simulink model "rx"  (R2019a)
settings: Solver=VariableStepAuto  StartTime=0.0  StopTime=10.0  RelTol=1e-3
undefined symbols (not defined in the file): fdesignblkfcn, gcbh
libraries: audiosources x1
settings Model: Creator=vicda  LastModifiedBy=vicda

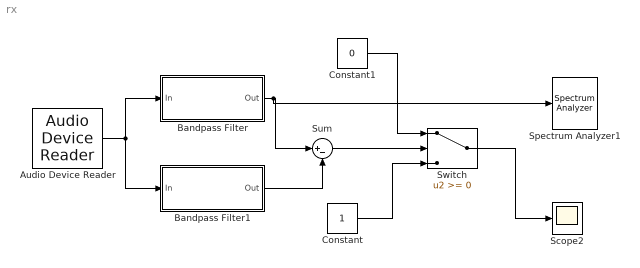
== system rx ==
  Audio Device Reader : audiosources/Audio Device Reader  Driver=DirectSound  Device=Default  SampleRate=44100  NumChannels=1  SamplesPerFrame=512  BitDepth=16-bit integer  NumBuffers=10  DefaultInputChannelMapping=on  InputChannelMapping=1:2  OutputNumOverrunSamples=off  OutputDataType=double  DriverIdx=1  DeviceWarnFlag=''
      settings: SourceProductName=Audio Toolbox  SourceProductBaseCode=AU
  Bandpass Filter : Subsystem  DialogController=fdesignblkfcn  InitFcn=fdesignblkfcn(gcbh, {'InitFcn'});  mask(Bandpass Filter){}
      mask help: Design a bandpass filter
      settings: CopyFcn=fdesignblkfcn(gcbh, {'CopyFcn'});
      mask Help: helpview(mapfilelocation('dsp'), 'dspbandpassfilter');
      mask Display: disp('Bandpass');
  Bandpass Filter1 : Subsystem  DialogController=fdesignblkfcn  InitFcn=fdesignblkfcn(gcbh, {'InitFcn'});  mask(Bandpass Filter){}
      mask help: Design a bandpass filter
      settings: CopyFcn=fdesignblkfcn(gcbh, {'CopyFcn'});
      mask Help: helpview(mapfilelocation('dsp'), 'dspbandpassfilter');
      mask Display: disp('Bandpass');
  Constant : Constant
  Constant1 : Constant  Value=0
  Scope2 : Scope
  Spectrum Analyzer1 : SpectrumAnalyzer
  Sum : Sum  Inputs=|+-
  Switch : Switch
  wires:
  Audio Device Reader/1 -> Bandpass Filter1/1(In), Bandpass Filter/1(In)
  Sum/1 -> Switch/2
  Constant/1 -> Switch/3
  Constant1/1 -> Switch/1
  Switch/1 -> Scope2/1
  Bandpass Filter/1(Out) -> Spectrum Analyzer1/1, Sum/1
  Bandpass Filter1/1(Out) -> Sum/2

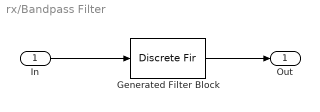
== system rx/Bandpass Filter ==
  In : Inport
  Generated Filter Block : DiscreteFir  Tag=BlockMethodSubSystem  Coefficients=[-0.000434773882586315453 -0.00807784253181313694 0.0237316368736724195 -0.0179551613016422189 -0.00559013199008739914 -0.00293522567996073189 0.0204369862189881547 0.0273874115135967697 -0.0729941141400381049 0.0225736738416546165 -0.0242724714232191857 0.175036757677766969 -0.162534911455741088 -0.196323384054438721 0.443315559598018272 -0.196323384054438721 -0.162534911455741088 0.175036757677766969 -0.0242724714232191857 0.0225736738416546165 -0.0729941141400381049 0.0273874115135967697 0.0204369862189881547 -0.00293522567996073189 -0.00559013199008739914 -0.0179551613016422189 0.0237316368736724195 -0.00807784253181313694 -0.000434773882586315453]  InputProcessing=Columns as channels (frame based)
  Out : Outport
  wires:
  In/1 -> Generated Filter Block/1
  Generated Filter Block/1 -> Out/1

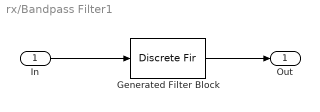
== system rx/Bandpass Filter1 ==
  In : Inport
  Generated Filter Block : DiscreteFir  Tag=BlockMethodSubSystem  Coefficients=[0.0021076805989375543 -0.00404438869893899988 0.00264259349110617953 0.00339189165923243184 -0.00921932481510973761 0.00822936574471131062 -0.00128829099518638218 -0.00221806756386821839 -0.00310982952279529115 0.00774902945952622713 0.00316117944458285671 -0.0268236848239911257 0.038168816285184648 -0.0181351136958959464 -0.0170561195013439748 0.0297795993752242687 -0.0103079521309629579 -0.00221246633346986951 -0.0325561067738429077 0.0896906667413850667 -0.0862162505231355708 -0.0241828892916038651 0.172770850425035483 -0.221172816433308106 0.101263760164629069 0.101263760164629069 -0.221172816433308106 0.172770850425035483 -0.0241828892916038651 -0.0862162505231355708 0.0896906667413850667 -0.0325561067738429077 -0.00221246633346986951 -0.0103079521309629579 0.0297795993752242687 -0.0170561195013439748 -0.0181351136958959464 0.038168816285184648 -0.0268236848239911257 0.00316117944458285671 0.00774902945952622713 -0.00310982952279529115 -0.00221806756386821839 -0.00128829099518638218 0.00822936574471131062 -0.00921932481510973761 0.00339189165923243184 0.00264259349110617953 -0.00404438869893899988 0.0021076805989375543]  InputProcessing=Columns as channels (frame based)
  Out : Outport
  wires:
  In/1 -> Generated Filter Block/1
  Generated Filter Block/1 -> Out/1
